simulink library "AEMS_Standard_Library"  (R2016b)
(part 14 of 39)

      mask TypeOptions LibType: _DGNTRP | _DGNOK
      mask Display:
      | dgn_mask = ['Event ID: ' char(EventId) '\n Library type: ' char(LibType)];
      | 
      | disp(dgn_mask);
      | plot([5,5,5])
      | plot([6,6,6])
  AEMS_DEM_SET_STORAGE_COND_1D : Subsystem  Tag=[LIB]  mask(AEMS_DEM_SET_STORAGE_COND_1D){StorageCondId=Dem_StorageConditionId_XXX}
      mask prompts: StorageCondId "Storage Condition Id :"
      mask init:
      | eval([char(StorageCondId) ' = 0;']);
      | 
      | storagecond_b1 = find_system(gcb,'LookUnderMasks','all','FollowLinks','on','Name','StorageCondId_block');
      | 
      | set_param([storagecond_b1{:}],'Value',[char(StorageCondId)]);
      settings: AttributesFormatString=%<MaskType>\nStorage Condition Id : = %<StorageCondId>
      mask Display:
      | port_label('input',1,'conditionfulfilled');
      | 
      | dgn_mask = char(StorageCondId);
      | 
      | disp(dgn_mask);
      | 
      | plot([5,5,5])
      | plot([6,6,6])
  AEMS_DEM_SET_STORAGE_COND_2D : Subsystem  Tag=[LIB]  mask(AEMS_DEM_SET_STORAGE_COND_2D){StorageCondId=Dem_StorageConditionId_XXX}
      mask prompts: StorageCondId "Storage Condition Id :"
      mask init:
      | lib_path = gcb;
      | StorageCond_Id=get_param(lib_path,'StorageCondId');
      | storagecond_b1 = find_system(lib_path,'LookUnderMasks','all','FollowLinks','on','Name','StorageConditionId_block1');
      | eval([char(StorageCond_Id) '= 0;']);
      | set_param(storagecond_b1{:},'Value',char(StorageCond_Id));
      | storagecond_b = find_system(lib_path,'LookUnderMasks','all','FollowLinks','on','regexp','on','Name','^StorageConditionId_block');
      | for len=2:length(storagecond_b)
      | Splitname=regexp(StorageCond_Id,'_','all');
      | storageCondId=insertBefore(StorageCond_Id,Splitname(end),num2str(len));
      | eval([char(storageCondId) '= 0;']);
      | set_param(storagecond_b{len},'Value',char(storageCondId));
      | end
      | 
      | % set_param([encond_b1{:}],'Value',[char(StorageCondId) '_1']);
      | % set_param([encond_b2{:}],'Value',[char(StorageCondId) '_2']);
      settings: AttributesFormatString=%<MaskType>\nStorage Condition Id : = %<StorageCondId>
      mask Display:
      | port_label('input',1,'conditionfulfilled');
      | 
      | dgn_mask = char(StorageCondId);
      | 
      | disp(dgn_mask);
      | 
      | plot([5,5,5])
      | plot([6,6,6])
  AEMS_DEM_SET_STORAGE_COND_8D : Subsystem  Tag=[LIB]  mask(AEMS_DEM_SET_STORAGE_COND_8D){StorageCondId=Dem_StorageConditionId_XXX}
      mask prompts: StorageCondId "Storage Condition Id :"
      mask init:
      | % eval([char(StorageCondId) '_1 = 0;']);
      | % eval([char(StorageCondId) '_2 = 0;']);
      | % eval([char(StorageCondId) '_3 = 0;']);
      | % eval([char(StorageCondId) '_4 = 0;']);
      | % eval([char(StorageCondId) '_5 = 0;']);
      | % eval([char(StorageCondId) '_6 = 0;']);
      | % eval([char(StorageCondId) '_7 = 0;']);
      | % eval([char(StorageCondId) '_8 = 0;']);
      | 
      | lib_path = gcb;
      | StorageCond_Id=get_param(lib_path,'StorageCondId');
      | encond_b1 = find_system(lib_path,'LookUnderMasks','all','FollowLinks','on','Name','StorageConditionId_block1');
      | eval([char(StorageCond_Id) '= 0;']);
      | set_param(encond_b1{:},'Value',char(StorageCond_Id));
      | storagecond_b = find_system(lib_path,'LookUnderMasks','all','FollowLinks','on','regexp','on','Name','^StorageConditionId_block');
      | for len=2:length(storagecond_b)
      | Splitname=regexp(StorageCond_Id,'_','all');
      | storageCondId=insertBefore(StorageCond_Id,Splitname(end),num2str(len));
      | eval([char(storageCondId) '= 0;']);
      | set_param(storagecond_b{len},'Value',char(storageCondId));
      | end
      | 
      | % storagecond_b1 = find_system(gcb,'LookUnderMasks','all','FollowLinks','on','Name','StorageConditionId_block1');
      | % storagecond_b2 = find_system(gcb,'LookUnderMasks','all','FollowLinks','on','Name','StorageConditionId_block2');
      | % storagecond_b3 = find_system(gcb,'LookUnderMasks','all','FollowLinks','on','Name','StorageConditionId_block3');
      | % storagecond_b4 = find_system(gcb,'LookUnderMasks','all','FollowLinks','on','Name','StorageConditionId_block4');
      | % storagecond_b5 = find_system(gcb,'LookUnderMasks','all','FollowLinks','on','Name','StorageConditionId_block5');
      | % storagecond_b6 = find_system(gcb,'LookUnderMasks','all','FollowLinks','on','Name','StorageConditionId_block6');
      | % storagecond_b7 = find_system(gcb,'LookUnderMasks','all','FollowLinks','on','Name','StorageConditionId_block7');
      | % storagecond_b8 = find_system(gcb,'LookUnderMasks','all','FollowLinks','on','Name','StorageConditionId_block8');
      | % 
      | % set_param([storagecond_b1{:}],'Value',[char(StorageCondId) '_1']);
      | % set_param([storagecond_b2{:}],'Value',[char(StorageCondId) '_2']);
      | % set_param([storagecond_b3{:}],'Value',[char(StorageCondId) '_3']);
      | % set_param([storagecond_b4{:}],'Value',[char(StorageCondId) '_4']);
      | % set_param([storagecond_b5{:}],'Value',[char(StorageCondId) '_5']);
      | % set_param([storagecond_b6{:}],'Value',[char(StorageCondId) '_6']);
      | % set_param([storagecond_b7{:}],'Value',[char(StorageCondId) '_7']);
      | % set_param([storagecond_b8{:}],'Value',[char(StorageCondId) '_8']);
      settings: AttributesFormatString=%<MaskType>\nStorage Condition Id : = %<StorageCondId>
      mask Display:
      | port_label('input',1,'conditionfulfilled');
      | 
      | dgn_mask = char(StorageCondId);
      | 
      | disp(dgn_mask);
      | 
      | plot([5,5,5])
      | plot([6,6,6])
  AEMS_DEM_TIMEBASEDDEBOUNCE : Subsystem  Tag=[LIB]  mask(AEMS_DEM_TIMEBASEDDEBOUNCE){eventid=Dem_EventId, sampletime=0.01}
      mask prompts: eventid "Identifier of a diagnostic event (EventID)"; sampletime "Sample Time"
      mask help:
      | It  transmit the status Failed or Passed to the DEM. Accordingly,
      | some bits of the UDS DTC status byte changes synchronously or
      | asynchronously according to the configuration.
      |
      | -INPUTS-
      | conditionfulfilled: specifies whether the storage condition assigned
      | to the StorageConditionID is fulfilled
      | prefailed: Monitor reports nonqualified test result pre-failed
      | prepassed: Monitor reports nonqualified test result pre-passed
      | reseteventdebounce: Freeze or reset the internal debounce timer.
      |
      | -OUTPUTS-
      | debouncevalue_for_failed: Value of debounce when an event failed
      | debouncevalue_for_passed: Value of debounce when an event passed
      | failed: Diagnostic monitor reports an event failed
      | passed: Diagnostic monitor reports an event passed
      |
      | -PARAMETERS-
      | EventID: Internal identifier of a diagnostic event. 0 is not a valid value.
      | Debounce Behavior: The event debounce counter will be frozen or reset
      | (0 for FREEZE and 1 for RESET)
      | Debounce Time Failed Threshold: Defines the time out duration for
      | "Event Failed" qualification.
      | Debounce Time Passed Threshold: Defines the time out duration for
      | "Event Passed" qualification.
      mask init:
      | eval([char(eventid) '= 0;'])
      | 
      | eventid_b = find_system(gcb,'LookUnderMasks','all','FollowLinks','on','Name','EventId_block');
      | set_param([eventid_b{:}],'Value',char(eventid));
      | 
      | try
      |     set_param([gcb,'/Subsystem_Timer_Debounce_Call/AEMS_TIMER_H1'],'sample_time',sampletime);
      |     set_param([gcb,'/Subsystem_Timer_Debounce_Call/AEMS_TIMER_H'],'sample_time',sampletime);
      | end
      settings: AttributesFormatString=|
      | %<MaskType>
      | EventId: %<eventid>
      | Sample time: %<sampletime>
      mask TypeOptions sampletime: 0.001 | 0.002 | 0.004 | 0.01 | 0.02 | 0.1
  AEMS_DEM_TIME_BASED_DEBOUNCE_1D : Subsystem  Tag=[LIB]  Description=This subsystem is interface for self diagnosis standard calculated from similar condition and NG judgment.  mask(AEMS_DEM_TIME_BASED_DEBOUNCE_1D){eventid=Dem_EventId_Device_Faulttype, DemDebounceBehavior1=DEM_DEBOUNCE_FREEZE (0), DemDebounceTimeFailedThreshold=Cxx_dem_fail_thd_Device_Faulttype, DemDebounceTimePassedThreshold=Cxx_dem_pass_thd_Device_Faulttype, DemTimeBypassFailure=Cbx_dem_byp_fail_Device_Faulttype, Sample_Time=0.01}
      mask prompts: eventid "Identifier of a diagnostic event (EventId)"; DemDebounceBehavior1 "Dem Debounce Behavior"; DemDebounceTimeFailedThreshold "Dem Debounce Time Failed Threshold"; DemDebounceTimePassedThreshold "Dem Debounce Time Passed Threshold"; DemTimeBypassFailure "Dem Debounce Time Bypass Failure"
      mask help:
      | It  transmit the status Failed or Passed to the DEM. Accordingly,
      | some bits of the UDS DTC status byte changes synchronously or
      | asynchronously according to the configuration.
      |
      | -INPUTS-
      | conditionfulfilled: specifies whether the storage condition assigned
      | to the StorageConditionID is fulfilled
      | prefailed: Monitor reports nonqualified test result pre-failed
      | prepassed: Monitor reports nonqualified test result pre-passed
      | reseteventdebounce: Freeze or reset the internal debounce timer.
      |
      | -OUTPUTS-
      | debouncevalue_for_failed: Value of debounce when an event failed
      | debouncevalue_for_passed: Value of debounce when an event passed
      | failed: Diagnostic monitor reports an event failed
      | passed: Diagnostic monitor reports an event passed
      |
      | -PARAMETERS-
      | EventID: Internal identifier of a diagnostic event. 0 is not a valid value.
      | Debounce Behavior: The event debounce counter will be frozen or reset
      | (0 for FREEZE and 1 for RESET)
      | Debounce Time Failed Threshold: Defines the time out duration for
      | "Event Failed" qualification.
      | Debounce Time Passed Threshold: Defines the time out duration for
      | "Event Passed" qualification.
      mask init:
      | ThisBlk =gcb;
      | behaviorblk = [ThisBlk,'/DemDebounceBehavior'];
      | Bpath = [ThisBlk,'/AEMS_DEM_TIME_BASED_DEBOUNCE_CALL/AEMS_DEM_TIMEBASEDDEBOUNCE'];
      | set_param(Bpath,'eventid',eventid);
      | if strcmpi(DemDebounceBehavior1,'DEM_DEBOUNCE_FREEZE (0)')
      |    set_param(behaviorblk,'Value','0');
      | elseif strcmpi(DemDebounceBehavior1,'DEM_DEBOUNCE_RESET (1)')
      |     set_param(behaviorblk,'Value','1');
      | end
      | set_param([ThisBlk,'/AEMS_DEM_TIME_BASED_DEBOUNCE_CALL/AEMS_DEM_TIMEBASEDDEBOUNCE'],'sampletime',Sample_Time);
      settings: AttributesFormatString=|
      | %<MaskType>
      | EventId: %<eventid>\nDem Debounce Behavior = %<DemDebounceBehavior1>\nDem Debounce Time Failed Threshold = %<DemDebounceTimeFailedThreshold>\nDem Debounce Time Passed Threshold = %<DemDebounceTimePassedThreshold>\nDem Debounce Time Bypass Failure = %<DemTimeBypassFailure>\nSample_Time = %<Sample_Time>
      mask Help:
      | eval('path_lib=fileparts(which(''AEMS_Standard_Library''));');
      | doc_path = [path_lib '\help\AEMS_DEM_TIME_BASED_DEBOUNCE.pdf'];
      | eval('open(doc_path)')
      mask TypeOptions DemDebounceBehavior1: DEM_DEBOUNCE_FREEZE (0) | DEM_DEBOUNCE_RESET (1)
      mask TypeOptions Sample_Time: 0.001 | 0.002 | 0.004 | 0.01 | 0.02 | 0.1
  AEMS_DEM_TIME_BASED_DEBOUNCE_2D : Subsystem  Tag=[LIB]  Description=This subsystem is interface for self diagnosis standard calculated from similar condition and NG judgment.  mask(AEMS_DEM_TIME_BASED_DEBOUNCE_2D){eventid=Dem_EventId_Device_Faulttype, DemDebounceBehavior1=DEM_DEBOUNCE_FREEZE (0), DemDebounceBehavior2=DEM_DEBOUNCE_FREEZE (0), DemDebounceTimeFailedThreshold=Cxx_dem_fail_thd_Device_Faulttype, DemDebounceTimePassedThreshold=Cxx_dem_pass_thd_Device_Faulttype, DemTimeBypassFailure=Cbx_dem_byp_fail_Device_Faulttype, Sample_Time=0.01}
      mask prompts: eventid "Identifier of a diagnostic event (EventId)"; DemDebounceBehavior1 "Dem Debounce Behavior 1"; DemDebounceBehavior2 "Dem Debounce Behavior 2"; DemDebounceTimeFailedThreshold "Dem Debounce Time Failed Threshold"; DemDebounceTimePassedThreshold "Dem Debounce Time Passed Threshold"; DemTimeBypassFailure "Dem Debounce Time Bypass Failure"
      mask help:
      | It  transmit the status Failed or Passed to the DEM. Accordingly,
      | some bits of the UDS DTC status byte changes synchronously or
      | asynchronously according to the configuration.
      |
      | -INPUTS-
      | conditionfulfilled: specifies whether the storage condition assigned
      | to the StorageConditionID is fulfilled
      | prefailed: Monitor reports nonqualified test result pre-failed
      | prepassed: Monitor reports nonqualified test result pre-passed
      | reseteventdebounce: Freeze or reset the internal debounce timer.
      |
      | -OUTPUTS-
      | debouncevalue_for_failed: Value of debounce when an event failed
      | debouncevalue_for_passed: Value of debounce when an event passed
      | failed: Diagnostic monitor reports an event failed
      | passed: Diagnostic monitor reports an event passed
      |
      | -PARAMETERS-
      | EventID: Internal identifier of a diagnostic event. 0 is not a valid value.
      | Debounce Behavior: The event debounce counter will be frozen or reset
      | (0 for FREEZE and 1 for RESET)
      | Debounce Time Failed Threshold: Defines the time out duration for
      | "Event Failed" qualification.
      | Debounce Time Passed Threshold: Defines the time out duration for
      | "Event Passed" qualification.
      mask init:
      | ThisBlk =gcb;
      | DemDebounceBehaviors = {DemDebounceBehavior1,DemDebounceBehavior2};   
      | behaviorblk = [ThisBlk,'/DemDebounceBehavior'];
      | behaviorvector = '[';
      |     for cnt=1:2        
      |         cnt_str=num2str(cnt);
      |         Bpath = [ThisBlk,'/AEMS_DEM_TIME_BASED_DEBOUNCE_CALL',cnt_str,'/AEMS_DEM_TIMEBASEDDEBOUNCE'];
      | %         set_param(Bpath,'eventid',[eventid,'_' cnt_str]);
      |         if (cnt==1)
      |             set_param(Bpath,'eventid',eventid);
      |         else
      |             Splitname=regexp(eventid,'_','all');
      |             New_EventId=insertBefore(eventid,Splitname(end),num2str(cnt));
      |             set_param(Bpath,'eventid',New_EventId);
      |         end
      |         set_param(Bpath,'sampletime',Sample_Time);
      |         if strcmpi(DemDebounceBehaviors{cnt},'DEM_DEBOUNCE_FREEZE (0)')
      |            behaviorvector= [behaviorvector,'0,'];
      |         else    
      |            behaviorvector= [behaviorvector,'1,'];        
      |         end
      |     end
      |     behaviorvector = behaviorvector(1:end-1);%Why end-1? I want to skip ',' for the last field.
      |     behaviorvector = [behaviorvector,']'];
      |     set_param(behaviorblk,'Value',behaviorvector);
      settings: AttributesFormatString=|
      | %<MaskType>
      | EventId: %<eventid>\nDem Debounce Behavior 1 = %<DemDebounceBehavior1>\nDem Debounce Behavior 2 = %<DemDebounceBehavior2>\nDem Debounce Time Failed Threshold = %<DemDebounceTimeFailedThreshold>\nDem Debounce Time Passed Threshold = %<DemDebounceTimePassedThreshold>\nDem Debounce Time Bypass Failure = %<DemTimeBypassFailure>\nSample_Time = %<Sample_Time>
      mask Help:
      | eval('path_lib=fileparts(which(''AEMS_Standard_Library''));');
      | doc_path = [path_lib '\help\AEMS_DEM_TIME_BASED_DEBOUNCE.pdf'];
      | eval('open(doc_path)')
      mask TypeOptions DemDebounceBehavior1: DEM_DEBOUNCE_FREEZE (0) | DEM_DEBOUNCE_RESET (1)
      mask TypeOptions DemDebounceBehavior2: DEM_DEBOUNCE_FREEZE (0) | DEM_DEBOUNCE_RESET (1)
      mask TypeOptions Sample_Time: 0.001 | 0.002 | 0.004 | 0.01 | 0.02 | 0.1
  AEMS_DEM_TIME_BASED_DEBOUNCE_3D : Subsystem  Tag=[LIB]  Description=This subsystem is interface for self diagnosis standard calculated from similar condition and NG judgment.  mask(AEMS_DEM_TIME_BASED_DEBOUNCE_3D){eventid=Dem_EventId_Device_Faulttype, DemDebounceBehavior1=DEM_DEBOUNCE_FREEZE (0), DemDebounceBehavior2=DEM_DEBOUNCE_FREEZE (0), DemDebounceBehavior3=DEM_DEBOUNCE_FREEZE (0), DemDebounceTimeFailedThreshold=Cxx_dem_fail_thd_Device_Faulttype, DemDebounceTimePassedThreshold=Cxx_dem_pass_thd_Device_Faulttype, DemTimeBypassFailure=Cbx_dem_byp_fail_Device_Faulttype, Sample_Time=0.1}
      mask prompts: eventid "Identifier of a diagnostic event (EventId)"; DemDebounceBehavior1 "Dem Debounce Behavior 1"; DemDebounceBehavior2 "Dem Debounce Behavior 2"; DemDebounceBehavior3 "Dem Debounce Behavior 3"; DemDebounceTimeFailedThreshold "Dem Debounce Time Failed Threshold"; DemDebounceTimePassedThreshold "Dem Debounce Time Passed Threshold"; DemTimeBypassFailure "Dem Debounce Time Bypass Failure"
      mask help:
      | It  transmit the status Failed or Passed to the DEM. Accordingly,
      | some bits of the UDS DTC status byte changes synchronously or
      | asynchronously according to the configuration.
      |
      | -INPUTS-
      | conditionfulfilled: specifies whether the storage condition assigned
      | to the StorageConditionID is fulfilled
      | prefailed: Monitor reports nonqualified test result pre-failed
      | prepassed: Monitor reports nonqualified test result pre-passed
      | reseteventdebounce: Freeze or reset the internal debounce timer.
      |
      | -OUTPUTS-
      | debouncevalue_for_failed: Value of debounce when an event failed
      | debouncevalue_for_passed: Value of debounce when an event passed
      | failed: Diagnostic monitor reports an event failed
      | passed: Diagnostic monitor reports an event passed
      |
      | -PARAMETERS-
      | EventID: Internal identifier of a diagnostic event. 0 is not a valid value.
      | Debounce Behavior: The event debounce counter will be frozen or reset
      | (0 for FREEZE and 1 for RESET)
      | Debounce Time Failed Threshold: Defines the time out duration for
      | "Event Failed" qualification.
      | Debounce Time Passed Threshold: Defines the time out duration for
      | "Event Passed" qualification.
      mask init:
      | ThisBlk =gcb;
      | DemDebounceBehaviors = {DemDebounceBehavior1,DemDebounceBehavior2,DemDebounceBehavior3};  
      | behaviorblk = [ThisBlk,'/DemDebounceBehavior'];
      | behaviorvector = '[';
      |     for cnt=1:3        
      |         cnt_str=num2str(cnt);
      |         Bpath = [ThisBlk,'/AEMS_DEM_TIME_BASED_DEBOUNCE_CALL',cnt_str,'/AEMS_DEM_TIMEBASEDDEBOUNCE'];
      | %         set_param(Bpath,'eventid',[eventid,'_' cnt_str]);
      |         if (cnt==1)
      |             set_param(Bpath,'eventid',eventid);
      |         else
      |             Splitname=regexp(eventid,'_','all');
      |             New_EventId=insertBefore(eventid,Splitname(end),num2str(cnt));
      |             set_param(Bpath,'eventid',New_EventId);
      |         end
      |         set_param(Bpath,'sampletime',Sample_Time);
      |         if strcmpi(DemDebounceBehaviors{cnt},'DEM_DEBOUNCE_FREEZE (0)')
      |            behaviorvector= [behaviorvector,'0,'];
      |         else    
      |            behaviorvector= [behaviorvector,'1,'];        
      |         end
      |     end
      |     behaviorvector = behaviorvector(1:end-1);%Why end-1? I want to skip ',' for the last field.
      |     behaviorvector = [behaviorvector,']'];
      |     set_param(behaviorblk,'Value',behaviorvector);
      settings: AttributesFormatString=|
      | %<MaskType>
      | EventId: %<eventid>\nDem Debounce Behavior 1 = %<DemDebounceBehavior1>\nDem Debounce Behavior 2 = %<DemDebounceBehavior2>\nDem Debounce Behavior 3 = %<DemDebounceBehavior3>\nDem Debounce Time Failed Threshold = %<DemDebounceTimeFailedThreshold>\nDem Debounce Time Passed Threshold = %<DemDebounceTimePassedThreshold>\nDem Debounce Time Bypass Failure = %<DemTimeBypassFailure>\nSample_Time = %<Sample_Time>
      mask Help:
      | eval('path_lib=fileparts(which(''AEMS_Standard_Library''));');
      | doc_path = [path_lib '\help\AEMS_DEM_TIME_BASED_DEBOUNCE.pdf'];
      | eval('open(doc_path)')
      mask TypeOptions DemDebounceBehavior1: DEM_DEBOUNCE_FREEZE (0) | DEM_DEBOUNCE_RESET (1)
      mask TypeOptions DemDebounceBehavior2: DEM_DEBOUNCE_FREEZE (0) | DEM_DEBOUNCE_RESET (1)
      mask TypeOptions DemDebounceBehavior3: DEM_DEBOUNCE_FREEZE (0) | DEM_DEBOUNCE_RESET (1)
      mask TypeOptions Sample_Time: 0.001 | 0.002 | 0.004 | 0.01 | 0.02 | 0.1
  AEMS_DEM_TIME_BASED_DEBOUNCE_4D : Subsystem  Tag=[LIB]  Description=This subsystem is interface for self diagnosis standard calculated from similar condition and NG judgment.  mask(AEMS_DEM_TIME_BASED_DEBOUNCE_4D){eventid=Dem_EventId_Device_Faulttype, DemDebounceBehavior1=DEM_DEBOUNCE_FREEZE (0), DemDebounceBehavior2=DEM_DEBOUNCE_FREEZE (0), DemDebounceBehavior3=DEM_DEBOUNCE_FREEZE (0), DemDebounceBehavior4=DEM_DEBOUNCE_FREEZE (0), DemDebounceTimeFailedThreshold=Cxx_dem_fail_thd_Device_Faulttype, DemDebounceTimePassedThreshold=Cxx_dem_pass_thd_Device_Faulttype, DemTimeBypassFailure=Cbx_dem_byp_fail_Device_Faulttype, Sample_Time=0.01}
      mask prompts: eventid "Identifier of a diagnostic event (EventId)"; DemDebounceBehavior1 "Dem Debounce Behavior 1"; DemDebounceBehavior2 "Dem Debounce Behavior 2"; DemDebounceBehavior3 "Dem Debounce Behavior 3"; DemDebounceBehavior4 "Dem Debounce Behavior 4"; DemDebounceTimeFailedThreshold "Dem Debounce Time Failed Threshold"; DemDebounceTimePassedThreshold "Dem Debounce Time Passed Threshold"; DemTimeBypassFailure "Dem Debounce Time Bypass Failure"
      mask help:
      | It  transmit the status Failed or Passed to the DEM. Accordingly,
      | some bits of the UDS DTC status byte changes synchronously or
      | asynchronously according to the configuration.
      |
      | -INPUTS-
      | conditionfulfilled: specifies whether the storage condition assigned
      | to the StorageConditionID is fulfilled
      | prefailed: Monitor reports nonqualified test result pre-failed
      | prepassed: Monitor reports nonqualified test result pre-passed
      | reseteventdebounce: Freeze or reset the internal debounce timer.
      |
      | -OUTPUTS-
      | debouncevalue_for_failed: Value of debounce when an event failed
      | debouncevalue_for_passed: Value of debounce when an event passed
      | failed: Diagnostic monitor reports an event failed
      | passed: Diagnostic monitor reports an event passed
      |
      | -PARAMETERS-
      | EventID: Internal identifier of a diagnostic event. 0 is not a valid value.
      | Debounce Behavior: The event debounce counter will be frozen or reset
      | (0 for FREEZE and 1 for RESET)
      | Debounce Time Failed Threshold: Defines the time out duration for
      | "Event Failed" qualification.
      | Debounce Time Passed Threshold: Defines the time out duration for
      | "Event Passed" qualification.
      mask init:
      | ThisBlk =gcb;
      | DemDebounceBehaviors = {DemDebounceBehavior1,DemDebounceBehavior2,DemDebounceBehavior3,DemDebounceBehavior4};   
      | behaviorblk = [ThisBlk,'/DemDebounceBehavior'];
      | behaviorvector = '[';
      |     for cnt=1:4        
      |         cnt_str=num2str(cnt);
      |         Bpath = [ThisBlk,'/AEMS_DEM_TIME_BASED_DEBOUNCE_CALL',cnt_str,'/AEMS_DEM_TIMEBASEDDEBOUNCE'];
      | %         set_param(Bpath,'eventid',[eventid,'_' cnt_str]);
      |         if (cnt==1)
      |             set_param(Bpath,'eventid',eventid);
      |         else
      |             Splitname=regexp(eventid,'_','all');
      |             New_EventId=insertBefore(eventid,Splitname(end),num2str(cnt));
      |             set_param(Bpath,'eventid',New_EventId);
      |         end
      |         set_param(Bpath,'sampletime',Sample_Time);
      |         if strcmpi(DemDebounceBehaviors{cnt},'DEM_DEBOUNCE_FREEZE (0)')
      |            behaviorvector= [behaviorvector,'0,'];
      |         else    
      |            behaviorvector= [behaviorvector,'1,'];        
      |         end
      |     end
      |     behaviorvector = behaviorvector(1:end-1);%Why end-1? I want to skip ',' for the last field.
      |     behaviorvector = [behaviorvector,']'];
      |     set_param(behaviorblk,'Value',behaviorvector);
      settings: AttributesFormatString=|
      | %<MaskType>
      | EventId: %<eventid>\nDem Debounce Behavior 1 = %<DemDebounceBehavior1>\nDem Debounce Behavior 2 = %<DemDebounceBehavior2>\nDem Debounce Behavior 3 = %<DemDebounceBehavior3>\nDem Debounce Behavior 4 = %<DemDebounceBehavior4>\nDem Debounce Time Failed Threshold = %<DemDebounceTimeFailedThreshold>\nDem Debounce Time Passed Threshold = %<DemDebounceTimePassedThreshold>\nDem Debounce Time Bypass Failure = %<DemTimeBypassFailure>\nSample_Time = %<Sample_Time>
      mask Help:
      | eval('path_lib=fileparts(which(''AEMS_Standard_Library''));');
      | doc_path = [path_lib '\help\AEMS_DEM_TIME_BASED_DEBOUNCE.pdf'];
      | eval('open(doc_path)')
      mask TypeOptions DemDebounceBehavior1: DEM_DEBOUNCE_FREEZE (0) | DEM_DEBOUNCE_RESET (1)
      mask TypeOptions DemDebounceBehavior2: DEM_DEBOUNCE_FREEZE (0) | DEM_DEBOUNCE_RESET (1)
      mask TypeOptions DemDebounceBehavior3: DEM_DEBOUNCE_FREEZE (0) | DEM_DEBOUNCE_RESET (1)
      mask TypeOptions DemDebounceBehavior4: DEM_DEBOUNCE_FREEZE (0) | DEM_DEBOUNCE_RESET (1)
      mask TypeOptions Sample_Time: 0.001 | 0.002 | 0.004 | 0.01 | 0.02 | 0.1
  AEMS_DEM_TIME_BASED_DEBOUNCE_6D : Subsystem  Tag=[LIB]  Description=This subsystem is interface for self diagnosis standard calculated from similar condition and NG judgment.  mask(AEMS_DEM_TIME_BASED_DEBOUNCE_6D){eventid=Dem_EventId_Device_Faulttype, DemDebounceBehavior1=DEM_DEBOUNCE_FREEZE (0), DemDebounceBehavior2=DEM_DEBOUNCE_FREEZE (0), DemDebounceBehavior3=DEM_DEBOUNCE_FREEZE (0), DemDebounceBehavior4=DEM_DEBOUNCE_FREEZE (0), DemDebounceBehavior5=DEM_DEBOUNCE_FREEZE (0), DemDebounceBehavior6=DEM_DEBOUNCE_FREEZE (0), DemDebounceTimeFailedThreshold=Cxx_dem_fail_thd_Device_Faulttype, DemDebounceTimePassedThreshold=Cxx_dem_pass_thd_Device_Faulttype, DemTimeBypassFailure=Cbx_dem_byp_fail_Device_Faulttype, Sample_Time=0.01}
      mask prompts: eventid "Identifier of a diagnostic event (EventId)"; DemDebounceBehavior1 "Dem Debounce Behavior 1"; DemDebounceBehavior2 "Dem Debounce Behavior 2"; DemDebounceBehavior3 "Dem Debounce Behavior 3"; DemDebounceBehavior4 "Dem Debounce Behavior 4"; DemDebounceBehavior5 "Dem Debounce Behavior 5"; DemDebounceBehavior6 "Dem Debounce Behavior 6"; DemDebounceTimeFailedThreshold "Dem Debounce Time Failed Threshold"; DemDebounceTimePassedThreshold "Dem Debounce Time Passed Threshold"; DemTimeBypassFailure "Dem Debounce Time Bypass Failure"
      mask help:
      | It  transmit the status Failed or Passed to the DEM. Accordingly,
      | some bits of the UDS DTC status byte changes synchronously or
      | asynchronously according to the configuration.
      |
      | -INPUTS-
      | conditionfulfilled: specifies whether the storage condition assigned
      | to the StorageConditionID is fulfilled
      | prefailed: Monitor reports nonqualified test result pre-failed
      | prepassed: Monitor reports nonqualified test result pre-passed
      | reseteventdebounce: Freeze or reset the internal debounce timer.
      |
      | -OUTPUTS-
      | debouncevalue_for_failed: Value of debounce when an event failed
      | debouncevalue_for_passed: Value of debounce when an event passed
      | failed: Diagnostic monitor reports an event failed
      | passed: Diagnostic monitor reports an event passed
      |
      | -PARAMETERS-
      | EventID: Internal identifier of a diagnostic event. 0 is not a valid value.
      | Debounce Behavior: The event debounce counter will be frozen or reset
      | (0 for FREEZE and 1 for RESET)
      | Debounce Time Failed Threshold: Defines the time out duration for
      | "Event Failed" qualification.
      | Debounce Time Passed Threshold: Defines the time out duration for
      | "Event Passed" qualification.
      mask init:
      | ThisBlk =gcb;
      | DemDebounceBehaviors = {DemDebounceBehavior1,DemDebounceBehavior2,DemDebounceBehavior3,DemDebounceBehavior4,DemDebounceBehavior5,DemDebounceBehavior6};      
      | behaviorblk = [ThisBlk,'/DemDebounceBehavior'];
      | behaviorvector = '[';
      |     for cnt=1:6       
      |         cnt_str=num2str(cnt);
      |         Bpath = [ThisBlk,'/AEMS_DEM_TIME_BASED_DEBOUNCE_CALL',cnt_str,'/AEMS_DEM_TIMEBASEDDEBOUNCE'];
      | %         set_param(Bpath,'eventid',[eventid,'_' cnt_str]);
      |         if (cnt==1)
      |             set_param(Bpath,'eventid',eventid);
      |         else
      |             Splitname=regexp(eventid,'_','all');
      |             New_EventId=insertBefore(eventid,Splitname(end),num2str(cnt));
      |             set_param(Bpath,'eventid',New_EventId);
      |         end
      |         set_param(Bpath,'sampletime',Sample_Time);
      |         if strcmpi(DemDebounceBehaviors{cnt},'DEM_DEBOUNCE_FREEZE (0)')
      |            behaviorvector= [behaviorvector,'0,'];
      |         else    
      |            behaviorvector= [behaviorvector,'1,'];        
      |         end
      |     end
      |     behaviorvector = behaviorvector(1:end-1);%Why end-1? I want to skip ',' for the last field.
      |     behaviorvector = [behaviorvector,']'];
      |     set_param(behaviorblk,'Value',behaviorvector);
      settings: AttributesFormatString=|
      | %<MaskType>
      | EventId: %<eventid>\nDem Debounce Behavior 1 = %<DemDebounceBehavior1>\nDem Debounce Behavior 2 = %<DemDebounceBehavior2>\nDem Debounce Behavior 3 = %<DemDebounceBehavior3>\nDem Debounce Behavior 4 = %<DemDebounceBehavior4>\nDem Debounce Behavior 5 = %<DemDebounceBehavior5>\nDem Debounce Behavior 6 = %<DemDebounceBehavior6>\nDem Debounce Time Failed Threshold = %<DemDebounceTimeFailedThreshold>\nDem Debounce Time Passed Threshold = %<DemDebounceTimePassedThreshold>\nDem Debounce Time Bypass Failure = %<DemTimeBypassFailure>\nSample_Time = %<Sample_Time>
      mask Help:
      | eval('path_lib=fileparts(which(''AEMS_Standard_Library''));');
      | doc_path = [path_lib '\help\AEMS_DEM_TIME_BASED_DEBOUNCE.pdf'];
      | eval('open(doc_path)')
      mask TypeOptions DemDebounceBehavior1: DEM_DEBOUNCE_FREEZE (0) | DEM_DEBOUNCE_RESET (1)
      mask TypeOptions DemDebounceBehavior2: DEM_DEBOUNCE_FREEZE (0) | DEM_DEBOUNCE_RESET (1)
      mask TypeOptions DemDebounceBehavior3: DEM_DEBOUNCE_FREEZE (0) | DEM_DEBOUNCE_RESET (1)
      mask TypeOptions DemDebounceBehavior4: DEM_DEBOUNCE_FREEZE (0) | DEM_DEBOUNCE_RESET (1)
      mask TypeOptions DemDebounceBehavior5: DEM_DEBOUNCE_FREEZE (0) | DEM_DEBOUNCE_RESET (1)
      mask TypeOptions DemDebounceBehavior6: DEM_DEBOUNCE_FREEZE (0) | DEM_DEBOUNCE_RESET (1)
      mask TypeOptions Sample_Time: 0.001 | 0.002 | 0.004 | 0.01 | 0.02 | 0.1
  AEMS_DEM_TIME_BASED_DEBOUNCE_8D : Subsystem  Tag=[LIB]  Description=This subsystem is interface for self diagnosis standard calculated from similar condition and NG judgment.  mask(AEMS_DEM_TIME_BASED_DEBOUNCE_8D){eventid=Dem_EventId_Device_Faulttype, DemDebounceBehavior1=DEM_DEBOUNCE_FREEZE (0), DemDebounceBehavior2=DEM_DEBOUNCE_FREEZE (0), DemDebounceBehavior3=DEM_DEBOUNCE_FREEZE (0), DemDebounceBehavior4=DEM_DEBOUNCE_FREEZE (0), DemDebounceBehavior5=DEM_DEBOUNCE_FREEZE (0), DemDebounceBehavior6=DEM_DEBOUNCE_FREEZE (0), DemDebounceBehavior7=DEM_DEBOUNCE_FREEZE (0), DemDebounceBehavior8=DEM_DEBOUNCE_FREEZE (0), DemDebounceTimeFailedThreshold=Cxx_dem_fail_thd_Device_Faulttype, DemDebounceTimePassedThreshold=Cxx_dem_pass_thd_Device_Faulttype, DemTimeBypassFailure=Cbx_dem_byp_fail_Device_Faulttype, Sample_Time=0.01}
      mask prompts: eventid "Identifier of a diagnostic event (EventId)"; DemDebounceBehavior1 "Dem Debounce Behavior 1"; DemDebounceBehavior2 "Dem Debounce Behavior 2"; DemDebounceBehavior3 "Dem Debounce Behavior 3"; DemDebounceBehavior4 "Dem Debounce Behavior 4"; DemDebounceBehavior5 "Dem Debounce Behavior 5"; DemDebounceBehavior6 "Dem Debounce Behavior 6"; DemDebounceBehavior7 "Dem Debounce Behavior 7"; DemDebounceBehavior8 "Dem Debounce Behavior 8"; DemDebounceTimeFailedThreshold "Dem Debounce Time Failed Threshold"; DemDebounceTimePassedThreshold "Dem Debounce Time Passed Threshold"; DemTimeBypassFailure "Dem Debounce Time Bypass Failure"
      mask help:
      | It  transmit the status Failed or Passed to the DEM. Accordingly,
      | some bits of the UDS DTC status byte changes synchronously or
      | asynchronously according to the configuration.
      |
      | -INPUTS-
      | conditionfulfilled: specifies whether the storage condition assigned
      | to the StorageConditionID is fulfilled
      | prefailed: Monitor reports nonqualified test result pre-failed
      | prepassed: Monitor reports nonqualified test result pre-passed
      | reseteventdebounce: Freeze or reset the internal debounce timer.
      |
      | -OUTPUTS-
      | debouncevalue_for_failed: Value of debounce when an event failed
      | debouncevalue_for_passed: Value of debounce when an event passed
      | failed: Diagnostic monitor reports an event failed
      | passed: Diagnostic monitor reports an event passed
      |
      | -PARAMETERS-
      | EventID: Internal identifier of a diagnostic event. 0 is not a valid value.
      | Debounce Behavior: The event debounce counter will be frozen or reset
      | (0 for FREEZE and 1 for RESET)
      | Debounce Time Failed Threshold: Defines the time out duration for
      | "Event Failed" qualification.
      | Debounce Time Passed Threshold: Defines the time out duration for
      | "Event Passed" qualification.
      mask init:
      | ThisBlk =gcb;
      | DemDebounceBehaviors = {DemDebounceBehavior1,DemDebounceBehavior2,DemDebounceBehavior3,DemDebounceBehavior4,DemDebounceBehavior5,DemDebounceBehavior6,DemDebounceBehavior7,DemDebounceBehavior8};      
      | behaviorblk = [ThisBlk,'/DemDebounceBehavior'];
      | behaviorvector = '[';
      |     for cnt=1:8        
      |         cnt_str=num2str(cnt);
      |         Bpath = [ThisBlk,'/AEMS_DEM_TIME_BASED_DEBOUNCE_CALL',cnt_str,'/AEMS_DEM_TIMEBASEDDEBOUNCE'];
      | %         set_param(Bpath,'eventid',[eventid,'_' cnt_str]);
      |         if (cnt==1)
      |             set_param(Bpath,'eventid',eventid);
      |         else
      |             Splitname=regexp(eventid,'_','all');
      |             New_EventId=insertBefore(eventid,Splitname(end),num2str(cnt));
      |             set_param(Bpath,'eventid',New_EventId);
      |         end
      |         set_param(Bpath,'sampletime',Sample_Time);
      |         if strcmpi(DemDebounceBehaviors{cnt},'DEM_DEBOUNCE_FREEZE (0)')
      |            behaviorvector= [behaviorvector,'0,'];
      |         else    
      |            behaviorvector= [behaviorvector,'1,'];        
      |         end
      |     end
      |     behaviorvector = behaviorvector(1:end-1);%Why end-1? I want to skip ',' for the last field.
      |     behaviorvector = [behaviorvector,']'];
      |     set_param(behaviorblk,'Value',behaviorvector);
      | set_param(behaviorblk,'Value',behaviorvector);
      settings: AttributesFormatString=|
      | %<MaskType>
      | EventId: %<eventid>\nDem Debounce Behavior 1 = %<DemDebounceBehavior1>\nDem Debounce Behavior 2 = %<DemDebounceBehavior2>\nDem Debounce Behavior 3 = %<DemDebounceBehavior3>\nDem Debounce Behavior 4 = %<DemDebounceBehavior4>\nDem Debounce Behavior 5 = %<DemDebounceBehavior5>\nDem Debounce Behavior 6 = %<DemDebounceBehavior6>\nDem Debounce Behavior 7 = %<DemDebounceBehavior7>\nDem Debounce Behavior 8 = %<DemDebounceBehavior8>\nDem Debounce Time Failed Threshold = %<DemDebounceTimeFailedThreshold>\nDem Debounce Time Passed Threshold = %<DemDebounceTimePassedThreshold>\nDem Debounce Time Bypass Failure = %<DemTimeBypassFailure>\nSample_Time = %<Sample_Time>
      mask Help:
      | eval('path_lib=fileparts(which(''AEMS_Standard_Library''));');
      | doc_path = [path_lib '\help\AEMS_DEM_TIME_BASED_DEBOUNCE.pdf'];
      | eval('open(doc_path)')
      mask TypeOptions DemDebounceBehavior1: DEM_DEBOUNCE_FREEZE (0) | DEM_DEBOUNCE_RESET (1)
      mask TypeOptions DemDebounceBehavior2: DEM_DEBOUNCE_FREEZE (0) | DEM_DEBOUNCE_RESET (1)
      mask TypeOptions DemDebounceBehavior3: DEM_DEBOUNCE_FREEZE (0) | DEM_DEBOUNCE_RESET (1)
      mask TypeOptions DemDebounceBehavior4: DEM_DEBOUNCE_FREEZE (0) | DEM_DEBOUNCE_RESET (1)
      mask TypeOptions DemDebounceBehavior5: DEM_DEBOUNCE_FREEZE (0) | DEM_DEBOUNCE_RESET (1)
      mask TypeOptions DemDebounceBehavior6: DEM_DEBOUNCE_FREEZE (0) | DEM_DEBOUNCE_RESET (1)
      mask TypeOptions DemDebounceBehavior7: DEM_DEBOUNCE_FREEZE (0) | DEM_DEBOUNCE_RESET (1)
      mask TypeOptions DemDebounceBehavior8: DEM_DEBOUNCE_FREEZE (0) | DEM_DEBOUNCE_RESET (1)
      mask TypeOptions Sample_Time: 0.001 | 0.002 | 0.004 | 0.01 | 0.02 | 0.1
  AEMS_DEM_TIME_BASED_DEBOUNCE_THRSHOLD_DYN_1D : Subsystem  Tag=[LIB]  Description=This subsystem is interface for self diagnosis standard calculated from similar condition and NG judgment.  mask(AEMS_DEM_TIME_BASED_DEBOUNCE_THRSHOLD_DYN_1D){eventid=Dem_EventId_Device_Faulttype, DemDebounceBehavior1=DEM_DEBOUNCE_FREEZE (0), DemTimeBypassFailure=Cbx_dem_byp_fail_Device_Faulttype, Sample_Time=0.01}
      mask prompts: eventid "Identifier of a diagnostic event (EventId)"; DemDebounceBehavior1 "Dem Debounce Behavior"; DemTimeBypassFailure "Dem Debounce Time Bypass Failure"
      mask help:
      | It  transmit the status Failed or Passed to the DEM. Accordingly,
      | some bits of the UDS DTC status byte changes synchronously or
      | asynchronously according to the configuration.
      |
      | -INPUTS-
      | conditionfulfilled: specifies whether the storage condition assigned
      | to the StorageConditionID is fulfilled
      | prefailed: Monitor reports nonqualified test result pre-failed
      | prepassed: Monitor reports nonqualified test result pre-passed
      | reseteventdebounce: Freeze or reset the internal debounce timer.
      | failedthreshold: Defines the time out duration for
      | "Event Failed" qualification.
      | passedthreshold: Defines the time out duration for
      | "Event Passed" qualification.
      |
      | -OUTPUTS-
      | debouncevalue_for_failed: Value of debounce when an event failed
      | debouncevalue_for_passed: Value of debounce when an event passed
      | failed: Diagnostic monitor reports an event failed
      | passed: Diagnostic monitor reports an event passed
      |
      | -PARAMETERS-
      | EventID: Internal identifier of a diagnostic event. 0 is not a valid value.
      | Debounce Behavior: The event debounce counter will be frozen or reset
      | (0 for FREEZE and 1 for RESET)
      mask init:
      | ThisBlk =gcb;
      | behaviorblk = [ThisBlk,'/DemDebounceBehavior'];
      | Bpath = [ThisBlk,'/AEMS_DEM_TIME_BASED_DEBOUNCE_THRSHOLD_DYN_CALL/AEMS_DEM_TIMEBASEDDEBOUNCE'];
      | set_param(Bpath,'eventid',eventid);
      | if strcmpi(DemDebounceBehavior1,'DEM_DEBOUNCE_FREEZE (0)')
      |    set_param(behaviorblk,'Value','0');
      | elseif strcmpi(DemDebounceBehavior1,'DEM_DEBOUNCE_RESET (1)')
      |     set_param(behaviorblk,'Value','1');
      | end
      | set_param([ThisBlk,'/AEMS_DEM_TIME_BASED_DEBOUNCE_THRSHOLD_DYN_CALL/AEMS_DEM_TIMEBASEDDEBOUNCE'],'sampletime',Sample_Time);
      settings: AttributesFormatString=|
      | %<MaskType>
      | EventId: %<eventid>\nDem Debounce Behavior = %<DemDebounceBehavior1>\nDem Debounce Time Bypass Failure = %<DemTimeBypassFailure>\nSample_Time = %<Sample_Time>
      mask Help:
      | eval('path_lib=fileparts(which(''AEMS_Standard_Library''));');
      | doc_path = [path_lib '\help\AEMS_DEM_TIME_BASED_DEBOUNCE_THRSHOLD_DYN.pdf'];
      | eval('open(doc_path)')
      mask TypeOptions DemDebounceBehavior1: DEM_DEBOUNCE_FREEZE (0) | DEM_DEBOUNCE_RESET (1)
      mask TypeOptions Sample_Time: 0.001 | 0.002 | 0.004 | 0.01 | 0.02 | 0.1
  AEMS_DEM_TIME_BASED_DEBOUNCE_THRSHOLD_DYN_2D : Subsystem  Tag=[LIB]  Description=This subsystem is interface for self diagnosis standard calculated from similar condition and NG judgment.  mask(AEMS_DEM_TIME_BASED_DEBOUNCE_THRSHOLD_DYN_2D){eventid=Dem_EventId_Device_Faulttype, DemDebounceBehavior1=DEM_DEBOUNCE_FREEZE (0), DemDebounceBehavior2=DEM_DEBOUNCE_FREEZE (0), DemTimeBypassFailure=Cbx_dem_byp_fail_Device_Faulttype, Sample_Time=0.01}
      mask prompts: eventid "Identifier of a diagnostic event (EventId)"; DemDebounceBehavior1 "Dem Debounce Behavior 1"; DemDebounceBehavior2 "Dem Debounce Behavior 2"; DemTimeBypassFailure "Dem Debounce Time Bypass Failure"
      mask help:
      | It  transmit the status Failed or Passed to the DEM. Accordingly,
      | some bits of the UDS DTC status byte changes synchronously or
      | asynchronously according to the configuration.
      |
      | -INPUTS-
      | conditionfulfilled: specifies whether the storage condition assigned
      | to the StorageConditionID is fulfilled
      | prefailed: Monitor reports nonqualified test result pre-failed
      | prepassed: Monitor reports nonqualified test result pre-passed
      | reseteventdebounce: Freeze or reset the internal debounce timer.
      | failedthreshold: Defines the time out duration for
      | "Event Failed" qualification.
      | passedthreshold: Defines the time out duration for
      | "Event Passed" qualification.
      |
      | -OUTPUTS-
      | debouncevalue_for_failed: Value of debounce when an event failed
      | debouncevalue_for_passed: Value of debounce when an event passed
      | failed: Diagnostic monitor reports an event failed
      | passed: Diagnostic monitor reports an event passed
      |
      | -PARAMETERS-
      | EventID: Internal identifier of a diagnostic event. 0 is not a valid value.
      | Debounce Behavior: The event debounce counter will be frozen or reset
      | (0 for FREEZE and 1 for RESET)
      mask init:
      | ThisBlk =gcb;
      | DemDebounceBehaviors = {DemDebounceBehavior1,DemDebounceBehavior2};   
      | behaviorblk = [ThisBlk,'/DemDebounceBehavior'];
      | behaviorvector = '[';
      |     for cnt=1:2        
      |         cnt_str=num2str(cnt);
      |         Bpath = [ThisBlk,'/AEMS_DEM_TIME_BASED_DEBOUNCE_THRSHOLD_DYN_CALL',cnt_str,'/AEMS_DEM_TIMEBASEDDEBOUNCE'];
      | %         set_param(Bpath,'eventid',[eventid,'_' cnt_str]);
      |         if (cnt==1)
      |             set_param(Bpath,'eventid',eventid);
      |         else
      |             Splitname=regexp(eventid,'_','all');
      |             New_EventId=insertBefore(eventid,Splitname(end),num2str(cnt));
      |             set_param(Bpath,'eventid',New_EventId);
      |         end
      |         set_param(Bpath,'sampletime',Sample_Time);
      |         if strcmpi(DemDebounceBehaviors{cnt},'DEM_DEBOUNCE_FREEZE (0)')
      |            behaviorvector= [behaviorvector,'0,'];
      |         else    
      |            behaviorvector= [behaviorvector,'1,'];        
      |         end
      |     end
      |     behaviorvector = behaviorvector(1:end-1);%Why end-1? I want to skip ',' for the last field.
      |     behaviorvector = [behaviorvector,']'];
      |     set_param(behaviorblk,'Value',behaviorvector);
      settings: AttributesFormatString=|
      | %<MaskType>
      | EventId: %<eventid>\nDem Debounce Behavior 1 = %<DemDebounceBehavior1>\nDem Debounce Behavior 2 = %<DemDebounceBehavior2>\nDem Debounce Time Bypass Failure = %<DemTimeBypassFailure>\nSample_Time = %<Sample_Time>
      mask Help:
      | eval('path_lib=fileparts(which(''AEMS_Standard_Library''));');
      | doc_path = [path_lib '\help\AEMS_DEM_TIME_BASED_DEBOUNCE_THRSHOLD_DYN.pdf'];
      | eval('open(doc_path)')
      mask TypeOptions DemDebounceBehavior1: DEM_DEBOUNCE_FREEZE (0) | DEM_DEBOUNCE_RESET (1)
      mask TypeOptions DemDebounceBehavior2: DEM_DEBOUNCE_FREEZE (0) | DEM_DEBOUNCE_RESET (1)
      mask TypeOptions Sample_Time: 0.001 | 0.002 | 0.004 | 0.01 | 0.02 | 0.1
  AEMS_DEM_TIME_BASED_DEBOUNCE_THRSHOLD_DYN_3D : Subsystem  Tag=[LIB]  Description=This subsystem is interface for self diagnosis standard calculated from similar condition and NG judgment.  mask(AEMS_DEM_TIME_BASED_DEBOUNCE_THRSHOLD_DYN_3D){eventid=Dem_EventId_Device_Faulttype, DemDebounceBehavior1=DEM_DEBOUNCE_FREEZE (0), DemDebounceBehavior2=DEM_DEBOUNCE_FREEZE (0), DemDebounceBehavior3=DEM_DEBOUNCE_FREEZE (0), DemTimeBypassFailure=Cbx_dem_byp_fail_Device_Faulttype, Sample_Time=0.01}
      mask prompts: eventid "Identifier of a diagnostic event (EventId)"; DemDebounceBehavior1 "Dem Debounce Behavior 1"; DemDebounceBehavior2 "Dem Debounce Behavior 2"; DemDebounceBehavior3 "Dem Debounce Behavior 3"; DemTimeBypassFailure "Dem Debounce Time Bypass Failure"
      mask help:
      | It  transmit the status Failed or Passed to the DEM. Accordingly,
      | some bits of the UDS DTC status byte changes synchronously or
      | asynchronously according to the configuration.
      |
      | -INPUTS-
      | conditionfulfilled: specifies whether the storage condition assigned
      | to the StorageConditionID is fulfilled
      | prefailed: Monitor reports nonqualified test result pre-failed
      | prepassed: Monitor reports nonqualified test result pre-passed
      | reseteventdebounce: Freeze or reset the internal debounce timer.
      | failedthreshold: Defines the time out duration for
      | "Event Failed" qualification.
      | passedthreshold: Defines the time out duration for
      | "Event Passed" qualification.
      |
      | -OUTPUTS-
      | debouncevalue_for_failed: Value of debounce when an event failed
      | debouncevalue_for_passed: Value of debounce when an event passed
      | failed: Diagnostic monitor reports an event failed
      | passed: Diagnostic monitor reports an event passed
      |
      | -PARAMETERS-
      | EventID: Internal identifier of a diagnostic event. 0 is not a valid value.
      | Debounce Behavior: The event debounce counter will be frozen or reset
      | (0 for FREEZE and 1 for RESET)
      mask init:
      | ThisBlk =gcb;
      | DemDebounceBehaviors = {DemDebounceBehavior1,DemDebounceBehavior2,DemDebounceBehavior3};   
      | behaviorblk = [ThisBlk,'/DemDebounceBehavior'];
      | behaviorvector = '[';
      |     for cnt=1:3       
      |         cnt_str=num2str(cnt);
      |         Bpath = [ThisBlk,'/AEMS_DEM_TIME_BASED_DEBOUNCE_THRSHOLD_DYN_CALL',cnt_str,'/AEMS_DEM_TIMEBASEDDEBOUNCE'];
      | %         set_param(Bpath,'eventid',[eventid,'_' cnt_str]);
      |         if (cnt==1)
      |             set_param(Bpath,'eventid',eventid);
      |         else
      |             Splitname=regexp(eventid,'_','all');
      |             New_EventId=insertBefore(eventid,Splitname(end),num2str(cnt));
      |             set_param(Bpath,'eventid',New_EventId);
      |         end
      |         set_param(Bpath,'sampletime',Sample_Time);
      |         if strcmpi(DemDebounceBehaviors{cnt},'DEM_DEBOUNCE_FREEZE (0)')
      |            behaviorvector= [behaviorvector,'0,'];
      |         else    
      |            behaviorvector= [behaviorvector,'1,'];        
      |         end
      |     end
      |     behaviorvector = behaviorvector(1:end-1);%Why end-1? I want to skip ',' for the last field.
      |     behaviorvector = [behaviorvector,']'];
      |     set_param(behaviorblk,'Value',behaviorvector);
      settings: AttributesFormatString=|
      | %<MaskType>
      | EventId: %<eventid>\nDem Debounce Behavior 1 = %<DemDebounceBehavior1>\nDem Debounce Behavior 2 = %<DemDebounceBehavior2>\nDem Debounce Behavior 3 = %<DemDebounceBehavior3>\nDem Debounce Time Bypass Failure = %<DemTimeBypassFailure>\nSample_Time = %<Sample_Time>
      mask Help:
      | eval('path_lib=fileparts(which(''AEMS_Standard_Library''));');
      | doc_path = [path_lib '\help\AEMS_DEM_TIME_BASED_DEBOUNCE_THRSHOLD_DYN.pdf'];
      | eval('open(doc_path)')
      mask TypeOptions DemDebounceBehavior1: DEM_DEBOUNCE_FREEZE (0) | DEM_DEBOUNCE_RESET (1)
      mask TypeOptions DemDebounceBehavior2: DEM_DEBOUNCE_FREEZE (0) | DEM_DEBOUNCE_RESET (1)
      mask TypeOptions DemDebounceBehavior3: DEM_DEBOUNCE_FREEZE (0) | DEM_DEBOUNCE_RESET (1)
      mask TypeOptions Sample_Time: 0.001 | 0.002 | 0.004 | 0.01 | 0.02 | 0.1
  AEMS_DEM_TIME_BASED_DEBOUNCE_THRSHOLD_DYN_4D : Subsystem  Tag=[LIB]  Description=This subsystem is interface for self diagnosis standard calculated from similar condition and NG judgment.  mask(AEMS_DEM_TIME_BASED_DEBOUNCE_THRSHOLD_DYN_4D){eventid=Dem_EventId_Device_Faulttype, DemDebounceBehavior1=DEM_DEBOUNCE_FREEZE (0), DemDebounceBehavior2=DEM_DEBOUNCE_FREEZE (0), DemDebounceBehavior3=DEM_DEBOUNCE_FREEZE (0), DemDebounceBehavior4=DEM_DEBOUNCE_FREEZE (0), DemTimeBypassFailure=Cbx_dem_byp_fail_Device_Faulttype, Sample_Time=0.01}
      mask prompts: eventid "Identifier of a diagnostic event (EventId)"; DemDebounceBehavior1 "Dem Debounce Behavior 1"; DemDebounceBehavior2 "Dem Debounce Behavior 2"; DemDebounceBehavior3 "Dem Debounce Behavior 3"; DemDebounceBehavior4 "Dem Debounce Behavior 4"; DemTimeBypassFailure "Dem Debounce Time Bypass Failure"
      mask help:
      | It  transmit the status Failed or Passed to the DEM. Accordingly,
      | some bits of the UDS DTC status byte changes synchronously or
      | asynchronously according to the configuration.
      |
      | -INPUTS-
      | conditionfulfilled: specifies whether the storage condition assigned
      | to the StorageConditionID is fulfilled
      | prefailed: Monitor reports nonqualified test result pre-failed
      | prepassed: Monitor reports nonqualified test result pre-passed
      | reseteventdebounce: Freeze or reset the internal debounce timer.
      | failedthreshold: Defines the time out duration for
      | "Event Failed" qualification.
      | passedthreshold: Defines the time out duration for
      | "Event Passed" qualification.
      |
      | -OUTPUTS-
      | debouncevalue_for_failed: Value of debounce when an event failed
      | debouncevalue_for_passed: Value of debounce when an event passed
      | failed: Diagnostic monitor reports an event failed
      | passed: Diagnostic monitor reports an event passed
      |
      | -PARAMETERS-
      | EventID: Internal identifier of a diagnostic event. 0 is not a valid value.
      | Debounce Behavior: The event debounce counter will be frozen or reset
      | (0 for FREEZE and 1 for RESET)
      mask init:
      | ThisBlk =gcb;
      | DemDebounceBehaviors = {DemDebounceBehavior1,DemDebounceBehavior2,DemDebounceBehavior3,DemDebounceBehavior4};   
      | behaviorblk = [ThisBlk,'/DemDebounceBehavior'];
      | behaviorvector = '[';
      |     for cnt=1:4       
      |         cnt_str=num2str(cnt);
      |         Bpath = [ThisBlk,'/AEMS_DEM_TIME_BASED_DEBOUNCE_THRSHOLD_DYN_CALL',cnt_str,'/AEMS_DEM_TIMEBASEDDEBOUNCE'];
      | %         set_param(Bpath,'eventid',[eventid,'_' cnt_str]);
      |         if (cnt==1)
      |             set_param(Bpath,'eventid',eventid);
      |         else
      |             Splitname=regexp(eventid,'_','all');
      |             New_EventId=insertBefore(eventid,Splitname(end),num2str(cnt));
      |             set_param(Bpath,'eventid',New_EventId);
      |         end
      |         set_param(Bpath,'sampletime',Sample_Time);
      |         if strcmpi(DemDebounceBehaviors{cnt},'DEM_DEBOUNCE_FREEZE (0)')
      |            behaviorvector= [behaviorvector,'0,'];
      |         else    
      |            behaviorvector= [behaviorvector,'1,'];        
      |         end
      |     end
      |     behaviorvector = behaviorvector(1:end-1);%Why end-1? I want to skip ',' for the last field.
      |     behaviorvector = [behaviorvector,']'];
      |     set_param(behaviorblk,'Value',behaviorvector);
      settings: AttributesFormatString=|
      | %<MaskType>
      | EventId: %<eventid>\nDem Debounce Behavior 1 = %<DemDebounceBehavior1>\nDem Debounce Behavior 2 = %<DemDebounceBehavior2>\nDem Debounce Behavior 3 = %<DemDebounceBehavior3>\nDem Debounce Behavior 4 = %<DemDebounceBehavior4>\nDem Debounce Time Bypass Failure = %<DemTimeBypassFailure>\nSample_Time = %<Sample_Time>
      mask Help:
      | eval('path_lib=fileparts(which(''AEMS_Standard_Library''));');
      | doc_path = [path_lib '\help\AEMS_DEM_TIME_BASED_DEBOUNCE_THRSHOLD_DYN.pdf'];
      | eval('open(doc_path)')
      mask TypeOptions DemDebounceBehavior1: DEM_DEBOUNCE_FREEZE (0) | DEM_DEBOUNCE_RESET (1)
      mask TypeOptions DemDebounceBehavior2: DEM_DEBOUNCE_FREEZE (0) | DEM_DEBOUNCE_RESET (1)
      mask TypeOptions DemDebounceBehavior3: DEM_DEBOUNCE_FREEZE (0) | DEM_DEBOUNCE_RESET (1)
      mask TypeOptions DemDebounceBehavior4: DEM_DEBOUNCE_FREEZE (0) | DEM_DEBOUNCE_RESET (1)
      mask TypeOptions Sample_Time: 0.001 | 0.002 | 0.004 | 0.01 | 0.02 | 0.1
  AEMS_DEM_TIME_BASED_DEBOUNCE_THRSHOLD_DYN_6D : Subsystem  Tag=[LIB]  Description=This subsystem is interface for self diagnosis standard calculated from similar condition and NG judgment.  mask(AEMS_DEM_TIME_BASED_DEBOUNCE_THRSHOLD_DYN_6D){eventid=Dem_EventId_Device_Faulttype, DemDebounceBehavior1=DEM_DEBOUNCE_FREEZE (0), DemDebounceBehavior2=DEM_DEBOUNCE_FREEZE (0), DemDebounceBehavior3=DEM_DEBOUNCE_FREEZE (0), DemDebounceBehavior4=DEM_DEBOUNCE_FREEZE (0), DemDebounceBehavior5=DEM_DEBOUNCE_FREEZE (0), DemDebounceBehavior6=DEM_DEBOUNCE_FREEZE (0), DemTimeBypassFailure=Cbx_dem_byp_fail_Device_Faulttype, Sample_Time=0.01}
      mask prompts: eventid "Identifier of a diagnostic event (EventId)"; DemDebounceBehavior1 "Dem Debounce Behavior 1"; DemDebounceBehavior2 "Dem Debounce Behavior 2"; DemDebounceBehavior3 "Dem Debounce Behavior 3"; DemDebounceBehavior4 "Dem Debounce Behavior 4"; DemDebounceBehavior5 "Dem Debounce Behavior 5"; DemDebounceBehavior6 "Dem Debounce Behavior 6"; DemTimeBypassFailure "Dem Debounce Time Bypass Failure"
      mask help:
      | It  transmit the status Failed or Passed to the DEM. Accordingly,
      | some bits of the UDS DTC status byte changes synchronously or
      | asynchronously according to the configuration.
      |
      | -INPUTS-
      | conditionfulfilled: specifies whether the storage condition assigned
      | to the StorageConditionID is fulfilled
      | prefailed: Monitor reports nonqualified test result pre-failed
      | prepassed: Monitor reports nonqualified test result pre-passed
      | reseteventdebounce: Freeze or reset the internal debounce timer.
      | failedthreshold: Defines the time out duration for
      | "Event Failed" qualification.
      | passedthreshold: Defines the time out duration for
      | "Event Passed" qualification.
      |
      | -OUTPUTS-
      | debouncevalue_for_failed: Value of debounce when an event failed
      | debouncevalue_for_passed: Value of debounce when an event passed
      | failed: Diagnostic monitor reports an event failed
      | passed: Diagnostic monitor reports an event passed
      |
      | -PARAMETERS-
      | EventID: Internal identifier of a diagnostic event. 0 is not a valid value.
      | Debounce Behavior: The event debounce counter will be frozen or reset
      | (0 for FREEZE and 1 for RESET)
      mask init:
      | ThisBlk =gcb;
      | DemDebounceBehaviors = {DemDebounceBehavior1,DemDebounceBehavior2,DemDebounceBehavior3,DemDebounceBehavior4,DemDebounceBehavior5,DemDebounceBehavior6};   
      | behaviorblk = [ThisBlk,'/DemDebounceBehavior'];
      | behaviorvector = '[';
      |     for cnt=1:6      
      |         cnt_str=num2str(cnt);
      |         Bpath = [ThisBlk,'/AEMS_DEM_TIME_BASED_DEBOUNCE_THRSHOLD_DYN_CALL',cnt_str,'/AEMS_DEM_TIMEBASEDDEBOUNCE'];
      | %         set_param(Bpath,'eventid',[eventid,'_' cnt_str]);
      |         if (cnt==1)
      |             set_param(Bpath,'eventid',eventid);
      |         else
      |             Splitname=regexp(eventid,'_','all');
      |             New_EventId=insertBefore(eventid,Splitname(end),num2str(cnt));
      |             set_param(Bpath,'eventid',New_EventId);
      |         end
      |         set_param(Bpath,'sampletime',Sample_Time);
      |         if strcmpi(DemDebounceBehaviors{cnt},'DEM_DEBOUNCE_FREEZE (0)')
      |            behaviorvector= [behaviorvector,'0,'];
      |         else    
      |            behaviorvector= [behaviorvector,'1,'];        
      |         end
      |     end
      |     behaviorvector = behaviorvector(1:end-1);%Why end-1? I want to skip ',' for the last field.
      |     behaviorvector = [behaviorvector,']'];
      |     set_param(behaviorblk,'Value',behaviorvector);
      settings: AttributesFormatString=|
      | %<MaskType>
      | EventId: %<eventid>\nDem Debounce Behavior 1 = %<DemDebounceBehavior1>\nDem Debounce Behavior 2 = %<DemDebounceBehavior2>\nDem Debounce Behavior 3 = %<DemDebounceBehavior3>\nDem Debounce Behavior 4 = %<DemDebounceBehavior4>\nDem Debounce Behavior 5 = %<DemDebounceBehavior5>\nDem Debounce Behavior 6 = %<DemDebounceBehavior6>\nDem Debounce Time Bypass Failure = %<DemTimeBypassFailure>\nSample_Time = %<Sample_Time>
      mask Help:
      | eval('path_lib=fileparts(which(''AEMS_Standard_Library''));');
      | doc_path = [path_lib '\help\AEMS_DEM_TIME_BASED_DEBOUNCE_THRSHOLD_DYN.pdf'];
      | eval('open(doc_path)')
      mask TypeOptions DemDebounceBehavior1: DEM_DEBOUNCE_FREEZE (0) | DEM_DEBOUNCE_RESET (1)
      mask TypeOptions DemDebounceBehavior2: DEM_DEBOUNCE_FREEZE (0) | DEM_DEBOUNCE_RESET (1)
      mask TypeOptions DemDebounceBehavior3: DEM_DEBOUNCE_FREEZE (0) | DEM_DEBOUNCE_RESET (1)
      mask TypeOptions DemDebounceBehavior4: DEM_DEBOUNCE_FREEZE (0) | DEM_DEBOUNCE_RESET (1)
      mask TypeOptions DemDebounceBehavior5: DEM_DEBOUNCE_FREEZE (0) | DEM_DEBOUNCE_RESET (1)
      mask TypeOptions DemDebounceBehavior6: DEM_DEBOUNCE_FREEZE (0) | DEM_DEBOUNCE_RESET (1)
      mask TypeOptions Sample_Time: 0.001 | 0.002 | 0.004 | 0.01 | 0.02 | 0.1
  AEMS_DEM_TIME_BASED_DEBOUNCE_THRSHOLD_DYN_8D : Subsystem  Tag=[LIB]  Description=This subsystem is interface for self diagnosis standard calculated from similar condition and NG judgment.  mask(AEMS_DEM_TIME_BASED_DEBOUNCE_THRSHOLD_DYN_8D){eventid=Dem_EventId_Device_Faulttype, DemDebounceBehavior1=DEM_DEBOUNCE_FREEZE (0), DemDebounceBehavior2=DEM_DEBOUNCE_FREEZE (0), DemDebounceBehavior3=DEM_DEBOUNCE_FREEZE (0), DemDebounceBehavior4=DEM_DEBOUNCE_FREEZE (0), DemDebounceBehavior5=DEM_DEBOUNCE_FREEZE (0), DemDebounceBehavior6=DEM_DEBOUNCE_FREEZE (0), DemDebounceBehavior7=DEM_DEBOUNCE_FREEZE (0), DemDebounceBehavior8=DEM_DEBOUNCE_FREEZE (0), DemTimeBypassFailure=Cbx_dem_byp_fail_Device_Faulttype, Sample_Time=0.01}
      mask prompts: eventid "Identifier of a diagnostic event (EventId)"; DemDebounceBehavior1 "Dem Debounce Behavior 1"; DemDebounceBehavior2 "Dem Debounce Behavior 2"; DemDebounceBehavior3 "Dem Debounce Behavior 3"; DemDebounceBehavior4 "Dem Debounce Behavior 4"; DemDebounceBehavior5 "Dem Debounce Behavior 5"; DemDebounceBehavior6 "Dem Debounce Behavior 6"; DemDebounceBehavior7 "Dem Debounce Behavior 7"; DemDebounceBehavior8 "Dem Debounce Behavior 8"; DemTimeBypassFailure "Dem Debounce Time Bypass Failure"
      mask help:
      | It  transmit the status Failed or Passed to the DEM. Accordingly,
      | some bits of the UDS DTC status byte changes synchronously or
      | asynchronously according to the configuration.
      |
      | -INPUTS-
      | conditionfulfilled: specifies whether the storage condition assigned
      | to the StorageConditionID is fulfilled
      | prefailed: Monitor reports nonqualified test result pre-failed
      | prepassed: Monitor reports nonqualified test result pre-passed
      | reseteventdebounce: Freeze or reset the internal debounce timer.
      | failedthreshold: Defines the time out duration for
      | "Event Failed" qualification.
      | passedthreshold: Defines the time out duration for
      | "Event Passed" qualification.
      |
      | -OUTPUTS-
      | debouncevalue_for_failed: Value of debounce when an event failed
      | debouncevalue_for_passed: Value of debounce when an event passed
      | failed: Diagnostic monitor reports an event failed
      | passed: Diagnostic monitor reports an event passed
      |
      | -PARAMETERS-
      | EventID: Internal identifier of a diagnostic event. 0 is not a valid value.
      | Debounce Behavior: The event debounce counter will be frozen or reset
      | (0 for FREEZE and 1 for RESET)
      mask init:
      | ThisBlk =gcb;
      | DemDebounceBehaviors = {DemDebounceBehavior1,DemDebounceBehavior2,DemDebounceBehavior3,DemDebounceBehavior4,DemDebounceBehavior5,DemDebounceBehavior6,DemDebounceBehavior7,DemDebounceBehavior8};   
      | behaviorblk = [ThisBlk,'/DemDebounceBehavior'];
      | behaviorvector = '[';
      |     for cnt=1:8     
      |         cnt_str=num2str(cnt);
      |         Bpath = [ThisBlk,'/AEMS_DEM_TIME_BASED_DEBOUNCE_THRSHOLD_DYN_CALL',cnt_str,'/AEMS_DEM_TIMEBASEDDEBOUNCE'];
      | %         set_param(Bpath,'eventid',[eventid,'_' cnt_str]);
      |         if (cnt==1)
      |             set_param(Bpath,'eventid',eventid);
      |         else
      |             Splitname=regexp(eventid,'_','all');
      |             New_EventId=insertBefore(eventid,Splitname(end),num2str(cnt));
      |             set_param(Bpath,'eventid',New_EventId);
      |         end
      |         set_param(Bpath,'sampletime',Sample_Time);
      |         if strcmpi(DemDebounceBehaviors{cnt},'DEM_DEBOUNCE_FREEZE (0)')
      |            behaviorvector= [behaviorvector,'0,'];
      |         else    
      |            behaviorvector= [behaviorvector,'1,'];        
      |         end
      |     end
      |     behaviorvector = behaviorvector(1:end-1);%Why end-1? I want to skip ',' for the last field.
      |     behaviorvector = [behaviorvector,']'];
      |     set_param(behaviorblk,'Value',behaviorvector);
      settings: AttributesFormatString=|
      | %<MaskType>
      | EventId: %<eventid>\nDem Debounce Behavior 1 = %<DemDebounceBehavior1>\nDem Debounce Behavior 2 = %<DemDebounceBehavior2>\nDem Debounce Behavior 3 = %<DemDebounceBehavior3>\nDem Debounce Behavior 4 = %<DemDebounceBehavior4>\nDem Debounce Behavior 5 = %<DemDebounceBehavior5>\nDem Debounce Behavior 6 = %<DemDebounceBehavior6>\nDem Debounce Behavior 7 = %<DemDebounceBehavior7>\nDem Debounce Behavior 8 = %<DemDebounceBehavior8>\nDem Debounce Time Bypass Failure = %<DemTimeBypassFailure>\nSample_Time = %<Sample_Time>
      mask Help:
      | eval('path_lib=fileparts(which(''AEMS_Standard_Library''));');
      | doc_path = [path_lib '\help\AEMS_DEM_TIME_BASED_DEBOUNCE_THRSHOLD_DYN.pdf'];
      | eval('open(doc_path)')
      mask TypeOptions DemDebounceBehavior1: DEM_DEBOUNCE_FREEZE (0) | DEM_DEBOUNCE_RESET (1)
      mask TypeOptions DemDebounceBehavior2: DEM_DEBOUNCE_FREEZE (0) | DEM_DEBOUNCE_RESET (1)
      mask TypeOptions DemDebounceBehavior3: DEM_DEBOUNCE_FREEZE (0) | DEM_DEBOUNCE_RESET (1)
      mask TypeOptions DemDebounceBehavior4: DEM_DEBOUNCE_FREEZE (0) | DEM_DEBOUNCE_RESET (1)
      mask TypeOptions DemDebounceBehavior5: DEM_DEBOUNCE_FREEZE (0) | DEM_DEBOUNCE_RESET (1)
      mask TypeOptions DemDebounceBehavior6: DEM_DEBOUNCE_FREEZE (0) | DEM_DEBOUNCE_RESET (1)
      mask TypeOptions DemDebounceBehavior7: DEM_DEBOUNCE_FREEZE (0) | DEM_DEBOUNCE_RESET (1)
      mask TypeOptions DemDebounceBehavior8: DEM_DEBOUNCE_FREEZE (0) | DEM_DEBOUNCE_RESET (1)
      mask TypeOptions Sample_Time: 0.001 | 0.002 | 0.004 | 0.01 | 0.02 | 0.1
  AEMS_FIM_GETFUNCTIONPERMISSION : Subsystem  Tag=[LIB]  mask(AEMS_FIM_GETFUNCTIONPERMISSION){FID=Fim_fid_xxxx, FunctionMode=Functional}
      mask prompts: FID "Downgraded mode short name :"; FunctionMode "Function Mode"
      mask help:
      | This library calls AUTOSAR standard functions.
      | To know more details, please refer AUTOSAR FIM00011.
      mask init:
      | Thisblk = gcb;
      | Src_Of_Permission_Port = [Thisblk,'/Source_Of_Permission_Port'];
      | BlkType_Of_Source_Of_Permission_Port  = get_param(Src_Of_Permission_Port ,'BlockType');
      | 
      | if strcmp(FunctionMode,'Functional')
      |     if strcmp(BlkType_Of_Source_Of_Permission_Port  ,'Constant')
      |         %do nothing
      |     else
      |         if strcmp(BlkType_Of_Source_Of_Permission_Port  ,'Ground')
      |             replace_block(Src_Of_Permission_Port,'FollowLinks','on','BlockType','Ground','Constant','noprompt');
      |         else
      |             replace_block(Src_Of_Permission_Port,'FollowLinks','on','BlockType','DataStoreRead','Constant','noprompt');
      |         end
      |         set_param([Thisblk,'/Source_Of_Permission_Port'],'OutDataTypeStr','boolean');
      |     end
      |     
      | elseif strcmp(FunctionMode,'Dysfunctional')
      |     if strcmp(BlkType_Of_Source_Of_Permission_Port  ,'Ground')
      |         %do nothing
      |     else
      |         if strcmp(BlkType_Of_Source_Of_Permission_Port  ,'Constant')
      |             replace_block(Src_Of_Permission_Port,'FollowLinks','on','BlockType','Constant','Ground','noprompt');
      |         else
      |             replace_block(Src_Of_Permission_Port,'FollowLinks','on','BlockType','DataStoreRead','Ground','noprompt');
      |         end
      |     end
      |     
      | elseif strcmp(FunctionMode,'From Data Store memory')
      |     if strcmp(BlkType_Of_Source_Of_Permission_Port  ,'DataStoreRead')
      |         %do nothing
      |     else
      |         if strcmp(BlkType_Of_Source_Of_Permission_Port  ,'Constant')
      |             replace_block(Src_Of_Permission_Port,'FollowLinks','on','BlockType','Constant','DataStoreRead','noprompt');
      |         else
      |             replace_block(Src_Of_Permission_Port,'FollowLinks','on','BlockType','Ground','DataStoreRead','noprompt');
      |         end
      |     end
      |     %Get Task Rate of this block.(As per AEMS arch, all the blks shall be
      |     %kept under the runnable. The Runnable name will ncontain the sample
      |     %time suffix. From where we can get it.
      |     model_type_pos = strsplit(Thisblk,'/');%to split all the layer paths in order to get the runnable path
      |     runnable_path = [bdroot '/' model_type_pos{2}];%to get the runnable or AIPCALL path
      |     trg_port_name = get_param(find_system(runnable_path,'BlockType','TriggerPort'),'Name');%to get the function call trigger name
      |     TaskRate = '';%the raster suffix is stored in the parameter
      |     
      |     if ~isempty(trg_port_name)
      |         trg_port_name_spltd = strsplit(trg_port_name{1},'_');%splitting is done in order to get the raster and its type(Sched or Event)
      |         
      |         % checking for rasters of type Sched or Event especially occuring in
      |         % runnables
      |         if ~isempty(regexp(trg_port_name_spltd{1},'^Sched|^Event','once'))
      |             TaskRate = ['_' regexprep(trg_port_name_spltd{1},'Sched|Event','','once')];
      |             
      |             %checking if the raster is dcmcb and this is applicable only for
      |             %APICALL
      |         elseif ~isempty(regexp([trg_port_name_spltd{1} '_' trg_port_name_spltd{2} '_' ],'^DataServices_DCM_|^RoutineServices_DCM_','once'))||...
      |                 ~isempty(regexp(trg_port_name_spltd{1},'^Dcm$','once'))
      |             TaskRate = '_dcmcb';
      |             
      |             %checking if this block is used under the function call trigger
      |             %starting with "Com" and then giving an error message
      |             %this is applicable only for APICALL
      |         elseif ~isempty(regexp(trg_port_name_spltd{1},'^Com$','once'))
      |             msg = sprintf(['\n','The FIM block "' Thisblk '" should not be present within APICALLs having function call trigger as "Com"']);
      |             errordlg(msg);
      |             return;
      |         end
      |     end
      |     DataStoreName = [FID,TaskRate];
      | %     data_store_name = get_param([Thisblk,'/Source_Of_Permission_Port'],'DataStoreName');
      | %     if ~isequal(data_store_name,DataStoreName)
      |         set_param([Thisblk,'/Source_Of_Permission_Port'],'DataStoreName',DataStoreName);
      | %     end
      | end
      | % name_show = get_param([Thisblk,'/Source_Of_Permission_Port'],'ShowName');
      | % if isequal(name_show,'on')
      |     set_param([Thisblk,'/Source_Of_Permission_Port'],'ShowName','off');
      | % end
      settings: AttributesFormatString=%<MaskType>\nFunction Mode = %<FunctionMode>\nDowngraded mode short name : = %<FID>
      mask Help:
      | eval('path_lib=fileparts(which(''AEMS_Standard_Library''));');
      | mskblk=get_param(gcbh,'MaskType');
      | doc_path = [path_lib '\Help\',mskblk,'.pdf'];
      | eval('open(doc_path)');
      mask TypeOptions FunctionMode: Functional | Dysfunctional | From Data Store memory
      mask Display:
      | disp(['FiM_GetFunctionPermission \n \n \n \n \n']);
      | plot([5,5,5])
      | plot([6,6,6])
      | port_label('input',1,'FID')
      | port_label('output',1,'Permission')
      | %port_label('output',2,'FiM_Result')
  AEMS_FIM_GET_FUNC_PMT_1D : Subsystem  Tag=[LIB]  mask(AEMS_FIM_GET_FUNC_PMT_1D){FID=Fim_fid_xxxx, FunctionMode=Functional}
      mask prompts: FID "Downgraded mode short name :"; FunctionMode "Function Mode"
      mask help:
      | This library calls AUTOSAR standard functions.
      | To know more details, please refer AUTOSAR FIM00011.
      mask init:
      | libpath = gcb;
      | eval([char(FID) '= 0;'])
      | % Fid_b = find_system(libpath,'LookUnderMasks','all','FollowLinks','on','Name','FID_Block');
      | % child_lib_blk = find_system(libpath,'LookUnderMasks','all','FollowLinks','on','Name','AEMS_FIM_GETFUNCTIONPERMISSION');
      | set_param([gcb,'/FID_Block'],'Value',char(FID));
      | set_param([gcb,'/AEMS_FIM_GETFUNCTIONPERMISSION'],'FID',char(FID));
      | set_param([gcb,'/AEMS_FIM_GETFUNCTIONPERMISSION'],'FunctionMode',FunctionMode);
      settings: AttributesFormatString=%<MaskType>\nFunction Mode = %<FunctionMode>\nDowngraded mode short name : = %<FID>
      mask Help:
      | eval('path_lib=fileparts(which(''AEMS_Standard_Library''));');
      | mskblk=get_param(gcbh,'MaskType');
      | doc_path = [path_lib '\Help\',mskblk,'.pdf'];
      | eval('open(doc_path)');
      mask TypeOptions FunctionMode: Functional | Dysfunctional | From Data Store memory
      mask Display:
      | dgn_mask = ['Downgraded mode name  \n' char(FID)];
      | 
      | disp(dgn_mask);
      | plot([5,5,5])
      | plot([6,6,6])
  AEMS_FIM_GET_FUNC_PMT_2D : Subsystem  Tag=[LIB]  mask(AEMS_FIM_GET_FUNC_PMT_2D){FID=Fim_fid_xxxx, FunctionMode=Functional}
      mask prompts: FID "Downgraded mode short name :"; FunctionMode "Function Mode"
      mask help:
      | This library calls AUTOSAR standard functions.
      | To know more details, please refer AUTOSAR FIM00011.
      mask init:
      | This_Blk = gcb;
      | 
      | FID_1=[FID '_1'];
      | eval([char(FID_1) '= 0;']);
      | set_param([This_Blk,'/FID_Block1'],'Value',char(FID_1));
      | set_param([This_Blk,'/AEMS_FIM_GETFUNCTIONPERMISSION'],'FunctionMode',FunctionMode,'FID',FID_1);
      | 
      | FID_2=[FID '_2'];
      | eval([char(FID_2) '= 0;']);
      | set_param([This_Blk,'/FID_Block2'],'Value',char(FID_2));
      | set_param([This_Blk,'/AEMS_FIM_GETFUNCTIONPERMISSION1'],'FunctionMode',FunctionMode,'FID',FID_2);
      | 
      | % This_Blk = gcb;
      | % % eval([char(FID) '_1 = 0;'])
      | % % eval([char(FID) '_2 = 0;'])
      | % % Fid_b1 = find_system(gcb,'LookUnderMasks','all','FollowLinks','on','Name','FID_Block1');
      | % % Fid_b2 = find_system(gcb,'LookUnderMasks','all','FollowLinks','on','Name','FID_Block2');
      | % eval([char(FID) '= 0;']);
      | % set_param([This_Blk,'/FID_Block1'],'Value',FID);
      | % 
      | % Splitname=regexp(FID,'_','all');
      | % FID_2=insertBefore(FID,Splitname(end),num2str(2));
      | % eval([char(FID_2) '= 0;']);
      | % set_param([This_Blk,'/FID_Block2'],'Value',char(FID_2));
      | % 
      | % set_param([This_Blk,'/AEMS_FIM_GETFUNCTIONPERMISSION'],'FunctionMode',FunctionMode,'FID',FID);
      | % set_param([This_Blk,'/AEMS_FIM_GETFUNCTIONPERMISSION1'],'FunctionMode',FunctionMode,'FID',FID_2);
      settings: AttributesFormatString=%<MaskType>\nFunction Mode = %<FunctionMode>\nDowngraded mode short name : = %<FID>
      mask Help:
      | eval('path_lib=fileparts(which(''AEMS_Standard_Library''));');
      | mskblk=get_param(gcbh,'MaskType');
      | doc_path = [path_lib '\Help\',mskblk,'.pdf'];
      | eval('open(doc_path)');
      mask TypeOptions FunctionMode: Functional | Dysfunctional | From Data Store memory
      mask Display:
      | dgn_mask = ['Downgraded mode name \n' char(FID)];
      | 
      | disp(dgn_mask);
      | plot([5,5,5])
      | plot([6,6,6])
  AEMS_SORT_MEDIAN : Subsystem  Tag=[LIB]  mask(AEMS_SORT_MEDIAN){}
      mask help: To get the median vector after sorting the N numbers in ascending order.
      settings: AttributesFormatString=%<MaskType>
      mask Display: disp('AEMS_SORT_MEDIAN\n');
